simulink model "Go_to_goal2"  (R2025b)
settings: Solver=FixedStepAuto  StartTime=0.0  StopTime=inf  FixedStep=0.01  RelTol=1e-3  EnableMultiTasking=on
libraries: simulink x6, raspberrypiBasiclib x4, sensehatlib x1, raspberrypiNetworklib x1
settings Model: ExtModeTrigDuration=2  Creator=jujma  LastModifiedBy=jujma
settings SolverCC: PositivePriorityOrder=on
settings OptimizationCC: EnhancedBackFolding=on  PassReuseOutputArgsAs=Individual arguments  ZeroExternalMemoryAtStartup=off  ZeroInternalMemoryAtStartup=off  MaxStackSize=200000  OptimizeBlockOrder=speed  DifferentSizesBufferReuse=on  OptimizationCustomize=off  EfficientTunableParamExpr=on
settings DebuggingCC: ParameterTunabilityLossMsg=error
settings HardwareCC: ProdBitPerPointer=32.0  ProdBitPerSizeT=32.0  ProdBitPerPtrDiffT=32.0  ProdLargestAtomicInteger=Long  ProdLargestAtomicFloat=Double  ProdWordSize=32.0  ProdLongLongMode=on  ProdHWDeviceType=ARM Compatible->ARM Cortex-A (32-bit)
settings RTWCC: SystemTargetFile=ert.tlc  HardwareBoard=Raspberry Pi  TLCOptions="-aInlineSetEventsForThisBaseRateFcn=TLC_FALSE -aSuppressMultiTaskScheduler=TLC_FALSE  -aRateBasedStepFcn=0"  TemplateMakefile=ert_default_tmf  Toolchain=GNU GCC Embedded Linux  BuildConfiguration=Faster Runs  Description=Embedded Coder
settings CodeAppCC: ForceParamTrailComments=on  IgnoreCustomStorageClasses=off  OperatorAnnotations=on  SimulinkDataObjDesc=on  SFDataObjDesc=on  InsertBlockDesc=on
settings ERTTargetCC: ExtModeTransport=2.0  ExtModeStaticAlloc=on  ExtModeMexFile=ext_xcp  ExtModeIntrfLevel=Level2 - Open  InlinedParameterPlacement=Hierarchical  CodeReplacementLibrary=ARM Cortex-A CMSIS  SupportVariableSizeSignals=on

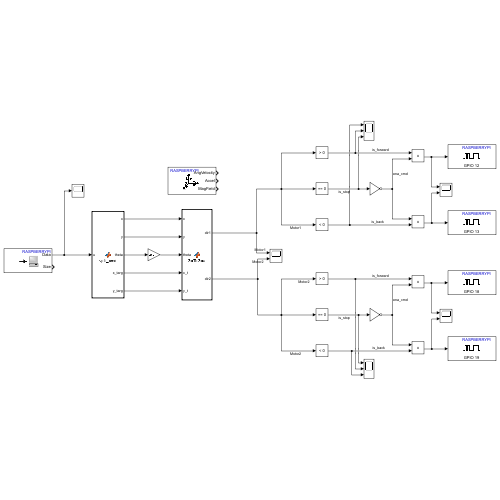
[thumbnail: Simulink's stored preview of the top-level diagram]
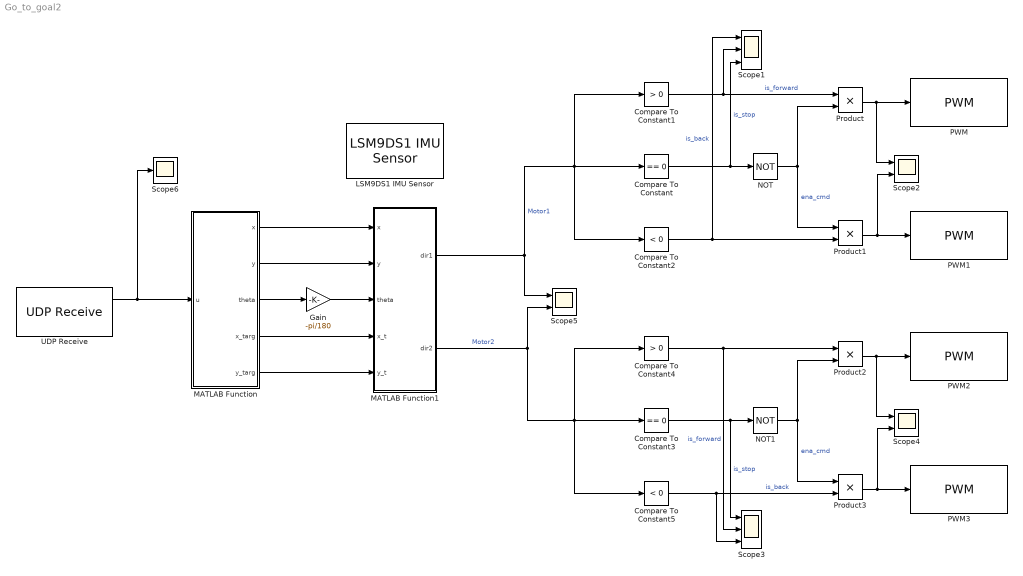
== system Go_to_goal2 ==
  Compare To Constant : simulink/Logic and Bit Operations/Compare To Constant  relop===  const=0  OutDataTypeStr=boolean
  Compare To Constant1 : simulink/Logic and Bit Operations/Compare To Constant  relop=>  const=0  OutDataTypeStr=boolean
  Compare To Constant2 : simulink/Logic and Bit Operations/Compare To Constant  relop=<  const=0  OutDataTypeStr=boolean
  Compare To Constant3 : simulink/Logic and Bit Operations/Compare To Constant  relop===  const=0  OutDataTypeStr=boolean
  Compare To Constant4 : simulink/Logic and Bit Operations/Compare To Constant  relop=>  const=0  OutDataTypeStr=boolean
  Compare To Constant5 : simulink/Logic and Bit Operations/Compare To Constant  relop=<  const=0  OutDataTypeStr=boolean
  Gain : Gain  Gain=-pi/180
  LSM9DS1 IMU Sensor : sensehatlib/LSM9DS1 IMU Sensor  blockPlatform=Raspberry Pi  BoardProperty_sh=Pi 3 Model B+  ActiveSensors_=Accelerometer, Gyroscope and Magnetometer  AccelerometerOutputDataRate=119 Hz  AccelerometerFullScaleRange=+/- 2g  AccelerometerBandwidth=50 Hz  GyroscopeOutputDataRate=119 Hz  GyroscopeFullScaleRange=245 dps  GyroscopeBandwidthMode=0  GyroscopeHighPassFilterEnabled=off  GyroscopeHighPassFilterMode=0  MagnetometerOutputDataRate=40 Hz  MagnetometerFullScaleRange=+/- 4 gauss  SampleTime=0.01
  MATLAB Function : MATLAB Function  TreatAsAtomicUnit=on
  MATLAB Function1 : MATLAB Function  TreatAsAtomicUnit=on
  NOT : Logic  Operator=NOT  IconShape=distinctive  AllPortsSameDT=off  OutDataTypeStr=boolean
  NOT1 : Logic  Operator=NOT  IconShape=distinctive  AllPortsSameDT=off  OutDataTypeStr=boolean
  PWM : raspberrypiBasiclib/PWM  board=Pi Zero W  Pin_=12  Frequency=500  blockPlatform=Raspberry Pi
  PWM1 : raspberrypiBasiclib/PWM  board=Pi Zero W  Pin_=13  Frequency=500  blockPlatform=Raspberry Pi
  PWM2 : raspberrypiBasiclib/PWM  board=Pi Zero W  Pin_=18  Frequency=500  blockPlatform=Raspberry Pi
  PWM3 : raspberrypiBasiclib/PWM  board=Pi Zero W  Pin_=19  Frequency=500  blockPlatform=Raspberry Pi
  Product{,1..3} (4 alike) : Product
  Scope1 : Scope  NumInputPorts=3
      settings: ActiveDisplayYMinimum=-0.12499999999999997  ActiveDisplayYMaximum=1.125  DataLoggingVariableName=ScopeData4
  Scope2 : Scope  NumInputPorts=2
      settings: ActiveDisplayYMinimum=-16.578406132891736  ActiveDisplayYMaximum=15.421593867108266
  Scope3 : Scope  NumInputPorts=3
      settings: ActiveDisplayYMinimum=-0.12499999999999997  ActiveDisplayYMaximum=1.125  DataLoggingVariableName=ScopeData2
  Scope4 : Scope  NumInputPorts=2
      settings: ActiveDisplayYMinimum=-16.578406132891736  ActiveDisplayYMaximum=15.421593867108266  DataLoggingVariableName=ScopeData3
  Scope5 : Scope  NumInputPorts=2
      settings: ActiveDisplayYMinimum=-1.25  ActiveDisplayYMaximum=1.25  DataLoggingVariableName=ScopeData5
  Scope6 : Scope
      settings: ActiveDisplayYMinimum=-1  ActiveDisplayYMaximum=1  DataLoggingVariableName=ScopeData6
  UDP Receive : raspberrypiNetworklib/UDP Receive  localURL='0.0.0.0'  localPort=50001  remoteURL='0.0.0.0'  remotePort=-1  recvBufferSize=8192  signalDatatype=double  dims=5  isVarSize=off  showBlockingTime=off  blockingTime=0  sampletime=0.01  blockPlatform=Raspberry Pi
  wires:
  Compare To Constant1/1 -> Scope1/2, Product/1  "is_forward"
  MATLAB Function1/2(dir2) -> Scope5/2, Compare To Constant4/1, Compare To Constant5/1, Compare To Constant3/1  "Motor2"
  Product1/1 -> Scope2/2, PWM1/1
  Compare To Constant/1 -> Scope1/3, NOT/1  "is_stop"
  NOT/1 -> Product/2, Product1/1  "ena_cmd"
  Compare To Constant4/1 -> Scope3/2, Product2/1  "is_forward"
  Product3/1 -> Scope4/2, PWM3/1
  Compare To Constant5/1 -> Scope3/3, Product3/2  "is_back"
  MATLAB Function1/1(dir1) -> Compare To Constant1/1, Compare To Constant2/1, Compare To Constant/1, Scope5/1  "Motor1"
  Compare To Constant3/1 -> Scope3/1, NOT1/1  "is_stop"
  Product2/1 -> Scope4/1, PWM2/1
  NOT1/1 -> Product2/2, Product3/1  "ena_cmd"
  Compare To Constant2/1 -> Scope1/1, Product1/2  "is_back"
  Product/1 -> Scope2/1, PWM/1
  UDP Receive/1 -> Scope6/1, MATLAB Function/1(u)
  MATLAB Function/4(x_targ) -> MATLAB Function1/4(x_t)
  MATLAB Function/1(x) -> MATLAB Function1/1(x)
  MATLAB Function/2(y) -> MATLAB Function1/2(y)
  MATLAB Function/3(theta) -> Gain/1
  MATLAB Function/5(y_targ) -> MATLAB Function1/5(y_t)
  Gain/1 -> MATLAB Function1/3(theta)

== matlab function Go_to_goal2/MATLAB Function1 ==
  data: x input; dir1 output; y input; theta input; x_t input; y_t input; dir2 output
function [dir1, dir2] = GoToGoal(x, y, theta, x_t, y_t)
% Discrete go-to-goal controller for differential drive.
% Outputs dir1, dir2 in {-1, 0, 1}.
%
% Behaviour:
%  - First: rotate in place until roughly facing target
%  - Then: drive forward while steering:
%       small error  -> [1 1]
%       medium error -> [0 1] or [1 0]  (arc turn)
%       large error  -> [-1 1] or [1 -1] (spin)

    % Vector to target and distance
    ex = x_t - x;
    ey = y_t - y;
    d  = sqrt(ex^2 + ey^2);

    % Persistent mode:
    % 1 = rotate to face target
    % 2 = drive + steer
    persistent mode
    if isempty(mode)
        mode = 1;
    end

    % Tolerances
    d_tol = 0.02;                 % stop radius (m)

    % Steering thresholds (tune these)
    face_tol   = 8  * pi/180;     % how well we must face target before driving
    steer_tol  = 6  * pi/180;     % below this, go straight
    spin_tol   = 25 * pi/180;     % above this, spin in place
    % Between steer_tol and spin_tol -> arc by stopping one wheel

    % Stop if close enough
    if d < d_tol
        dir1 = 0; dir2 = 0;
        mode = 1;
        return;
    end

    % Heading error to target
    psi     = atan2(ey, ex);
    e_theta = wrapToPi(psi - theta);

    % Decide turn direction:
    % e_theta > 0 => target is to the left => need CCW turn
    turnLeft = (e_theta > 0);

    switch mode
        case 1  % rotate in place until facing target (coarse alignment)
            if abs(e_theta) > face_tol
                if turnLeft
                    dir1 = -1; dir2 =  1;   % spin left (CCW)
                else
                    dir1 =  1; dir2 = -1;   % spin right (CW)
                end
            else
                mode = 2;
                dir1 = 1; dir2 = 1;        % start moving
            end

        case 2  % drive forward while steering
            if abs(e_theta) <= steer_tol
                % Close enough heading: go straight
                dir1 = 1; dir2 = 1;

            elseif abs(e_theta) >= spin_tol
                % Way off: spin in place to recover quickly
                if turnLeft
                    dir1 = -1; dir2 =  1;
                else
                    dir1 =  1; dir2 = -1;
                end

            else
                % Medium error: arc turn by stopping one wheel
                if turnLeft
                    % Need to turn left: slow/stop left wheel, keep right forward
                    dir1 = 0; dir2 = 1;     % arc left
                else
                    % Need to turn right: slow/stop right wheel, keep left forward
                    dir1 = 1; dir2 = 0;     % arc right
                end
            end

        otherwise
            dir1 = 0; dir2 = 0;
            mode = 1;
    end
end

function a = wrapToPi(a)
    a = mod(a + pi, 2*pi) - pi;
end

== matlab function Go_to_goal2/MATLAB Function ==
  data: u input; x output; y output; theta output; x_targ output; y_targ output
function [x, y, theta, x_targ, y_targ] = split_cmd(u)
%#codegen
% u is a 1x2 vector: [dir1 dir2]
x = u(1);
y = u(2);
theta = u(3);
x_targ = u(4);
y_targ = u(5);
end
